simulink model "sim_pos_dist_obs_tie"  (R2020a)
settings: Solver=ode4  StartTime=0.0  StopTime=30.0  FixedStep=0.01  RelTol=1e-3
values from neighbouring files (symbols this model uses):
  alfa_theta = 20    [init_pos_dist_obs_tie.m]
  alfa_theta_obs = 100    [init_pos_dist_obs_tie.m]
  beta1 = 1.2    [init_pos_dist_obs_tie.m]
  beta2 = 0.8    [init_pos_dist_obs_tie.m]
  delta_p_i_0 = zeros(3, NF)    [init_pos_dist_obs_tie.m]
  delta_v_i_0 = zeros(3, NF)    [init_pos_dist_obs_tie.m]
  dp_aa_t = 0.2 * ones(3, 5) + ( 1.0 - 0.2 ) * rand(3, 5)    [init_pos_dist_obs_tie.m]
  dp_ff_t = [ 0.4 * ones(1, 5) + ( 1.0 - 0.4 ) * rand(1, 5);                      0.4 * ones(1, 5) + ( 1.0 - 0.4 ) * rand(1, 5);                      0.2 * ones(1, 5) + ( 0.6 - 0.2 ) * rand(1, 5) ]    [init_pos_dist_obs_tie.m]
  dp_phi_t = ( - pi / 2 ) * ones(3, 5) + ( pi / 2 - ( - pi / 2 ) ) * rand(3, 5)    [init_pos_dist_obs_tie.m]
  ell1v = [2 * (Lv ^ (1/3)); 2 * (Lv ^ (1/3)); 2 * (Lv ^ (1/3))]    [init_pos_dist_obs_tie.m]
  ell2v = [1.5 * (Lv ^ (2/3)); 1.5 * (Lv ^ (2/3)); 1.5 * (Lv ^ (2/3))]    [init_pos_dist_obs_tie.m]
  ell3v = [1.1 * Lv; 1.1 * Lv; 1.1 * Lv]    [init_pos_dist_obs_tie.m]
  etai_0 = zeros(3,5)    [init_pos_dist_obs_tie.m]
  kai1v = [20; 20; 20]    [init_pos_dist_obs_tie.m]
  kai2v = [20; 20; 20]    [init_pos_dist_obs_tie.m]
  kai3v = [20; 20; 20]    [init_pos_dist_obs_tie.m]
  kai_1_t = 0.02    [init_pos_dist_obs_tie.m]
  kai_3_t = 0.1    [init_pos_dist_obs_tie.m]
  kai_chi_1 = diag([6; 6; 6])    [init_pos_dist_obs_tie.m]
  kai_chi_2 = diag([6; 6; 6])    [init_pos_dist_obs_tie.m]
  kai_u_1 = diag([8; 8; 8])    [init_pos_dist_obs_tie.m]
  kai_u_2 = diag([8; 8; 8])    [init_pos_dist_obs_tie.m]
  ksii_0 = zeros(3,5)    [init_pos_dist_obs_tie.m]
  l1v = diag([20; 20; 20])    [init_pos_dist_obs_tie.m]
  l2v = diag([30; 30; 30])    [init_pos_dist_obs_tie.m]
  mass_i = zeros(1,NF)    [init_pos_dist_obs_tie.m]
  Mii = diag([1;0;0;0;1])    [init_pos_dist_obs_tie.m]
  pos0 = zeros(3, 1)    [init_pos_dist_obs_tie.m]
  PZ0 = P0(3)    [init_pos_dist_obs_tie.m]
  PZ1 = 10    [init_pos_dist_obs_tie.m]
  Qci_init = repmat([1;0;0;0],1,NF)    [init_pos_dist_obs_tie.m]
  R0 = 4    [init_pos_dist_obs_tie.m]
  R1 = 8    [init_pos_dist_obs_tie.m]
  Rx2 = 10    [init_pos_dist_obs_tie.m]
  Ry2 = 6    [init_pos_dist_obs_tie.m]
  Rz2 = 4    [init_pos_dist_obs_tie.m]
  T0 = 0    [init_pos_dist_obs_tie.m]
  T1 = tseq1    (= 10)    [init_pos_dist_obs_tie.m]
  T12 = tseq1 + tseq12    (= 20)    [init_pos_dist_obs_tie.m]
  T2 = tseq1 + tseq12 + tseq2    (= 30)    [init_pos_dist_obs_tie.m]
  theta0 = ( 2 / 5 ) * pi    (= 1.25663706144)    [init_pos_dist_obs_tie.m]
  vel0 = zeros(3, 1)    [init_pos_dist_obs_tie.m]
  Wij = [0,0,1,0,0;              0,0,1,1,0;              1,0,0,0,1;              0,1,1,0,0;              0,0,1,0,0]    [init_pos_dist_obs_tie.m]
  X1 = 8    [init_pos_dist_obs_tie.m]
  X2 = 2    [init_pos_dist_obs_tie.m]
  X3 = 3    [init_pos_dist_obs_tie.m]
  Y1 = 10    [init_pos_dist_obs_tie.m]
  Y2 = 2    [init_pos_dist_obs_tie.m]
  Y3 = 4    [init_pos_dist_obs_tie.m]
  Z1 = 4    [init_pos_dist_obs_tie.m]
  Z2 = -6    [init_pos_dist_obs_tie.m]
  Z3 = 2    [init_pos_dist_obs_tie.m]
undefined symbols (not defined in the file or in its folder): cal_frac_squ, p_beta1, p_beta2, p_dbeta1, p_dbeta2, p_gamma1_pos, p_gamma1_vel, p_gamma2_pos, p_gamma2_vel, p_m_1, p_m_2, p_m_3, q_beta1, q_beta2, q_dbeta1, q_dbeta2, q_gamma1_pos, q_gamma1_vel, q_gamma2_pos, q_gamma2_vel, q_m_1, q_m_2, q_m_3
(part 4 of 4)

== matlab function sim_pos_dist_obs_tie/virtual velocity tracking item agent 1 ==
  data: kai_chi_1 input; chi_1 output; kai_chi_2 input; theta_err_ksi_1_vec input; theta_err_ksi_2_vec input
function chi_1 = fcn(kai_chi_1, kai_chi_2, theta_err_ksi_1_vec, theta_err_ksi_2_vec)
%%%% 固定时间虚拟速度控制量chi
iiuav = 1;
chi_1 = -kai_chi_1 * theta_err_ksi_1_vec(:,iiuav) - kai_chi_2 * theta_err_ksi_2_vec(:,iiuav);

== matlab function sim_pos_dist_obs_tie/virtual velocity tracking item agent 2 ==
  data: kai_chi_1 input; chi_2 output; kai_chi_2 input; theta_err_ksi_1_vec input; theta_err_ksi_2_vec input
function chi_2 = fcn(kai_chi_1, kai_chi_2, theta_err_ksi_1_vec, theta_err_ksi_2_vec)
%%%% 固定时间虚拟速度控制量chi
iiuav = 2;
chi_2 = -kai_chi_1 * theta_err_ksi_1_vec(:,iiuav) - kai_chi_2 * theta_err_ksi_2_vec(:,iiuav);

== matlab function sim_pos_dist_obs_tie/virtual velocity tracking item agent 3 ==
  data: kai_chi_1 input; chi_3 output; kai_chi_2 input; theta_err_ksi_1_vec input; theta_err_ksi_2_vec input
function chi_3 = fcn(kai_chi_1, kai_chi_2, theta_err_ksi_1_vec, theta_err_ksi_2_vec)
%%%% 固定时间虚拟速度控制量chi
iiuav = 3;
chi_3 = -kai_chi_1 * theta_err_ksi_1_vec(:,iiuav) - kai_chi_2 * theta_err_ksi_2_vec(:,iiuav);

== matlab function sim_pos_dist_obs_tie/virtual velocity tracking item agent 4 ==
  data: kai_chi_1 input; chi_4 output; kai_chi_2 input; theta_err_ksi_1_vec input; theta_err_ksi_2_vec input
function chi_4 = fcn(kai_chi_1, kai_chi_2, theta_err_ksi_1_vec, theta_err_ksi_2_vec)
%%%% 固定时间虚拟速度控制量chi
iiuav = 4;
chi_4 = -kai_chi_1 * theta_err_ksi_1_vec(:,iiuav) - kai_chi_2 * theta_err_ksi_2_vec(:,iiuav);

== matlab function sim_pos_dist_obs_tie/virtual velocity tracking item agent 5 ==
  data: kai_chi_1 input; chi_5 output; kai_chi_2 input; theta_err_ksi_1_vec input; theta_err_ksi_2_vec input
function chi_5 = fcn(kai_chi_1, kai_chi_2, theta_err_ksi_1_vec, theta_err_ksi_2_vec)
%%%% 固定时间虚拟速度控制量chi
iiuav = 5;
chi_5 = -kai_chi_1 * theta_err_ksi_1_vec(:,iiuav) - kai_chi_2 * theta_err_ksi_2_vec(:,iiuav);

== matlab function sim_pos_dist_obs_tie/combine chi ==
  data: chi_1 input; chi_2 input; chi_3 input; chi_4 input; chi_5 input; chi_vec output
function chi_vec  = fcn(chi_1, chi_2, chi_3, chi_4, chi_5)
%%%% 合并领导者位置观测器输出结果
chi_vec = [chi_1(:), chi_2(:), chi_3(:), chi_4(:), chi_5(:)];

== matlab function sim_pos_dist_obs_tie/generate translational disturbance agent 1 ==
  data: dp_aa_t input; dp_ff_t input; dp_phi_t input; dp_1 output; t input
function dp_1 = fcn(dp_aa_t, dp_ff_t, dp_phi_t, t)
%%%% 平移动力学方程中的扰动项设置
epsil_t = zeros(3, 1);

for kk = 1:5
    epsil_t = epsil_t + dp_aa_t(:, kk) .* sin( 2 * pi * dp_ff_t(:, kk) * t + dp_phi_t(:, kk) );
end

dp_1 = [ epsil_t(1) + 1.6 * sin( 0.4 * t ) + 2.0 * cos( 0.5 * t ) + 1.4 * sin( 0.7 * t ) ...
                + 4 * exp( -0.1 * t ) * sin( 0.8 * t ) + 3 / ( 1 + exp( -0.2 * ( t - 15 ) ) ); ...
                epsil_t(2) + 1.2 * sin( 0.2 * t ) + 3 * cos( 0.4 * t ) + 0.8 * sin( 0.6 * t ) ...
                + 2 * exp( -0.15 * t ) * cos( 1.2 * t ) + 3 / ( 1 + exp( -0.3 * ( t - 25 ) ) ); ...
                epsil_t(3) + 1.8 * sin( 0.2 * t ) + 1.6 * sin( 0.3 * t ) + 1.6 * cos( 0.4 * t ) ...
                + 4 * exp( -0.05 * t ) * sin( 0.5 * t + pi / 4 ) + 3 / ( 1 + exp( -0.5 * ( t - 20 ) ) ) ];

== matlab function sim_pos_dist_obs_tie/cal virtual velocity control error phi ==
  data: err_eta_vec input; chi_vec input; phi_vec output
function phi_vec  = fcn(err_eta_vec, chi_vec)
%%%% 合并领导者位置观测器输出结果
phi_vec = zeros(3,5);
for iiuav = 1:5
    phi_vec(:,iiuav) = err_eta_vec(:,iiuav) - chi_vec(:,iiuav);
end

== matlab function sim_pos_dist_obs_tie/cal abs 11 ==
  data: x input; y output
function y = fcn(x)
y = abs(x(:));

== matlab function sim_pos_dist_obs_tie/cal abs 12 ==
  data: x input; y output
function y = fcn(x)
y = abs(x(:));

== matlab function sim_pos_dist_obs_tie/choose ksi_est_err 11 ==
  data: x input; y output
function y = fcn(x)
iiuav = 1;
y = x(:,iiuav);

== matlab function sim_pos_dist_obs_tie/choose ksi_est_err 12 ==
  data: x input; y output
function y = fcn(x)
iiuav = 1;
y = x(:,iiuav);

== matlab function sim_pos_dist_obs_tie/trans to column10 ==
  data: x input; y output
function y = fcn(x)
y = x(:);

== matlab function sim_pos_dist_obs_tie/trans to column11 ==
  data: x input; y output
function y = fcn(x)
y = x(:);

== matlab function sim_pos_dist_obs_tie/cal d_theta_err_ksi agent 1 ==
  data: alfa_theta input; beta1 input; d_theta_err_ksi_1_1 output; beta2 input; d_err_ksi_squ_1_node_1 input; d_err_ksi_squ_2_node_1 input; err_ksi_squ_1_node_1 input; err_ksi_squ_2_node_1 input; err_ksi_vec input; d_theta_err_ksi_2_1 output; err_eta_vec input
function [d_theta_err_ksi_1_1, d_theta_err_ksi_2_1] = fcn(alfa_theta, beta1, beta2, d_err_ksi_squ_1_node_1, d_err_ksi_squ_2_node_1, ...
                                                                                                        err_ksi_squ_1_node_1, err_ksi_squ_2_node_1, err_ksi_vec, err_eta_vec)
%%%% 计算平滑递增函数的导数
iiuav = 1;
kk_alfa = alfa_theta;
d_theta_err_ksi_1_1 = ( beta1 .* d_err_ksi_squ_1_node_1(:) .* sign(err_ksi_vec(:,iiuav)) .* ( -1 + 2 ./ ( 1 + exp( -kk_alfa .* err_ksi_vec(:,iiuav) ) ) ) + ...
                                            err_ksi_squ_1_node_1(:) .* ( 2 .* kk_alfa .* exp( -kk_alfa .* err_ksi_vec(:,iiuav) ) ./ ( ( 1 + exp( -kk_alfa .* err_ksi_vec(:,iiuav) ) ) .^ 2) ) ) ...
                                            .* err_eta_vec(:,iiuav);
d_theta_err_ksi_2_1 = ( beta2 .* d_err_ksi_squ_2_node_1(:) .* sign(err_ksi_vec(:,iiuav)) .* ( -1 + 2 ./ ( 1 + exp( -kk_alfa .* err_ksi_vec(:,iiuav) ) ) ) + ...
                                            err_ksi_squ_2_node_1(:) .* ( 2 .* kk_alfa .* exp( -kk_alfa .* err_ksi_vec(:,iiuav) ) ./ ( ( 1 + exp( -kk_alfa .* err_ksi_vec(:,iiuav) ) ) .^ 2) ) ) ...
                                            .* err_eta_vec(:,iiuav);

== matlab function sim_pos_dist_obs_tie/cal abs 13 ==
  data: x input; y output
function y = fcn(x)
y = abs(x(:));

== matlab function sim_pos_dist_obs_tie/cal abs 14 ==
  data: x input; y output
function y = fcn(x)
y = abs(x(:));

== matlab function sim_pos_dist_obs_tie/cal d_theta_err_ksi agent 2 ==
  data: alfa_theta input; beta1 input; d_theta_err_ksi_1_2 output; beta2 input; d_err_ksi_squ_1_node_2 input; d_err_ksi_squ_2_node_2 input; err_ksi_squ_1_node_2 input; err_ksi_squ_2_node_2 input; err_ksi_vec input; d_theta_err_ksi_2_2 output; err_eta_vec input
function [d_theta_err_ksi_1_2, d_theta_err_ksi_2_2] = fcn(alfa_theta, beta1, beta2, d_err_ksi_squ_1_node_2, d_err_ksi_squ_2_node_2, ...
                                                                                                        err_ksi_squ_1_node_2, err_ksi_squ_2_node_2, err_ksi_vec, err_eta_vec)
%%%% 计算平滑递增函数的导数
iiuav = 2;
kk_alfa = alfa_theta;
d_theta_err_ksi_1_2 = ( beta1 .* d_err_ksi_squ_1_node_2(:) .* sign(err_ksi_vec(:,iiuav)) .* ( -1 + 2 ./ ( 1 + exp( -kk_alfa .* err_ksi_vec(:,iiuav) ) ) ) + ...
                                            err_ksi_squ_1_node_2(:) .* ( 2 .* kk_alfa .* exp( -kk_alfa .* err_ksi_vec(:,iiuav) ) ./ ( ( 1 + exp( -kk_alfa .* err_ksi_vec(:,iiuav) ) ) .^ 2) ) ) ...
                                            .* err_eta_vec(:,iiuav);
d_theta_err_ksi_2_2 = ( beta2 .* d_err_ksi_squ_2_node_2(:) .* sign(err_ksi_vec(:,iiuav)) .* ( -1 + 2 ./ ( 1 + exp( -kk_alfa .* err_ksi_vec(:,iiuav) ) ) ) + ...
                                            err_ksi_squ_2_node_2(:) .* ( 2 .* kk_alfa .* exp( -kk_alfa .* err_ksi_vec(:,iiuav) ) ./ ( ( 1 + exp( -kk_alfa .* err_ksi_vec(:,iiuav) ) ) .^ 2) ) ) ...
                                            .* err_eta_vec(:,iiuav);

== matlab function sim_pos_dist_obs_tie/generate translational disturbance agent 2 ==
  data: dp_aa_t input; dp_ff_t input; dp_phi_t input; dp_2 output; t input
function dp_2 = fcn(dp_aa_t, dp_ff_t, dp_phi_t, t)
%%%% 平移动力学方程中的扰动项设置
epsil_t = zeros(3, 1);

for kk = 1:5
    epsil_t = epsil_t + dp_aa_t(:, kk) .* sin( 2 * pi * dp_ff_t(:, kk) * t + dp_phi_t(:, kk) );
end

dp_2 = [ epsil_t(1) + 1.6 * sin( 0.2 * t ) + 2.0 * cos( 0.3 * t ) + 1.4 * sin( 0.5 * t ) ...
                + 4 * exp( -0.1 * t ) * sin( 0.5 * t ) + 3 / ( 1 + exp( -0.2 * ( t - 15 ) ) ); ...
                epsil_t(2) + 1.2 * sin( 0.1 * t ) + 3 * cos( 0.2 * t ) + 0.8 * sin( 0.4 * t ) ...
                + 2 * exp( -0.15 * t ) * cos( 0.6 * t ) + 3 / ( 1 + exp( -0.3 * ( t - 25 ) ) ); ...
                epsil_t(3) + 1.8 * sin( 0.1 * t ) + 1.6 * sin( 0.2 * t ) + 1.6 * cos( 0.3 * t ) ...
                + 4 * exp( -0.05 * t ) * sin( 0.4 * t + pi / 4 ) + 3 / ( 1 + exp( -0.5 * ( t - 20 ) ) ) ];

== matlab function sim_pos_dist_obs_tie/choose ksi_est_err 13 ==
  data: x input; y output
function y = fcn(x)
iiuav = 2;
y = x(:,iiuav);

== matlab function sim_pos_dist_obs_tie/choose ksi_est_err 14 ==
  data: x input; y output
function y = fcn(x)
iiuav = 2;
y = x(:,iiuav);

== matlab function sim_pos_dist_obs_tie/trans to column12 ==
  data: x input; y output
function y = fcn(x)
y = x(:);

== matlab function sim_pos_dist_obs_tie/trans to column13 ==
  data: x input; y output
function y = fcn(x)
y = x(:);

== matlab function sim_pos_dist_obs_tie/cal abs 15 ==
  data: x input; y output
function y = fcn(x)
y = abs(x(:));

== matlab function sim_pos_dist_obs_tie/cal abs 16 ==
  data: x input; y output
function y = fcn(x)
y = abs(x(:));

== matlab function sim_pos_dist_obs_tie/cal d_theta_err_ksi agent 3 ==
  data: alfa_theta input; beta1 input; d_theta_err_ksi_1_3 output; beta2 input; d_err_ksi_squ_1_node_3 input; d_err_ksi_squ_2_node_3 input; err_ksi_squ_1_node_3 input; err_ksi_squ_2_node_3 input; err_ksi_vec input; d_theta_err_ksi_2_3 output; err_eta_vec input
function [d_theta_err_ksi_1_3, d_theta_err_ksi_2_3] = fcn(alfa_theta, beta1, beta2, d_err_ksi_squ_1_node_3, d_err_ksi_squ_2_node_3, ...
                                                                                                        err_ksi_squ_1_node_3, err_ksi_squ_2_node_3, err_ksi_vec, err_eta_vec)
%%%% 计算平滑递增函数的导数
iiuav = 3;
kk_alfa = alfa_theta;
d_theta_err_ksi_1_3 = ( beta1 .* d_err_ksi_squ_1_node_3(:) .* sign(err_ksi_vec(:,iiuav)) .* ( -1 + 2 ./ ( 1 + exp( -kk_alfa .* err_ksi_vec(:,iiuav) ) ) ) + ...
                                            err_ksi_squ_1_node_3(:) .* ( 2 .* kk_alfa .* exp( -kk_alfa .* err_ksi_vec(:,iiuav) ) ./ ( ( 1 + exp( -kk_alfa .* err_ksi_vec(:,iiuav) ) ) .^ 2) ) ) ...
                                            .* err_eta_vec(:,iiuav);
d_theta_err_ksi_2_3 = ( beta2 .* d_err_ksi_squ_2_node_3(:) .* sign(err_ksi_vec(:,iiuav)) .* ( -1 + 2 ./ ( 1 + exp( -kk_alfa .* err_ksi_vec(:,iiuav) ) ) ) + ...
                                            err_ksi_squ_2_node_3(:) .* ( 2 .* kk_alfa .* exp( -kk_alfa .* err_ksi_vec(:,iiuav) ) ./ ( ( 1 + exp( -kk_alfa .* err_ksi_vec(:,iiuav) ) ) .^ 2) ) ) ...
                                            .* err_eta_vec(:,iiuav);

== matlab function sim_pos_dist_obs_tie/choose ksi_est_err 15 ==
  data: x input; y output
function y = fcn(x)
iiuav = 3;
y = x(:,iiuav);

== matlab function sim_pos_dist_obs_tie/choose ksi_est_err 16 ==
  data: x input; y output
function y = fcn(x)
iiuav = 3;
y = x(:,iiuav);

== matlab function sim_pos_dist_obs_tie/trans to column14 ==
  data: x input; y output
function y = fcn(x)
y = x(:);

== matlab function sim_pos_dist_obs_tie/trans to column15 ==
  data: x input; y output
function y = fcn(x)
y = x(:);

== matlab function sim_pos_dist_obs_tie/cal abs 17 ==
  data: x input; y output
function y = fcn(x)
y = abs(x(:));

== matlab function sim_pos_dist_obs_tie/cal abs 18 ==
  data: x input; y output
function y = fcn(x)
y = abs(x(:));

== matlab function sim_pos_dist_obs_tie/generate translational disturbance agent 3 ==
  data: dp_aa_t input; dp_ff_t input; dp_phi_t input; dp_3 output; t input
function dp_3 = fcn(dp_aa_t, dp_ff_t, dp_phi_t, t)
%%%% 平移动力学方程中的扰动项设置
epsil_t = zeros(3, 1);

for kk = 1:5
    epsil_t = epsil_t + dp_aa_t(:, kk) .* sin( 2 * pi * dp_ff_t(:, kk) * t + dp_phi_t(:, kk) );
end

dp_3 = [ epsil_t(1) + 1.6 * sin( 0.2 * t ) + 2.0 * cos( 0.3 * t ) + 1.4 * sin( 0.5 * t ) ...
                + 4 * exp( -0.1 * t ) * sin( 0.5 * t ) + 3 / ( 1 + exp( -0.2 * ( t - 15 ) ) ); ...
                epsil_t(2) + 1.2 * sin( 0.1 * t ) + 3 * cos( 0.2 * t ) + 0.8 * sin( 0.4 * t ) ...
                + 2 * exp( -0.15 * t ) * cos( 0.6 * t ) + 3 / ( 1 + exp( -0.3 * ( t - 25 ) ) ); ...
                epsil_t(3) + 1.8 * sin( 0.1 * t ) + 1.6 * sin( 0.2 * t ) + 1.6 * cos( 0.3 * t ) ...
                + 4 * exp( -0.05 * t ) * sin( 0.4 * t + pi / 4 ) + 3 / ( 1 + exp( -0.5 * ( t - 20 ) ) ) ];

== matlab function sim_pos_dist_obs_tie/cal d_theta_err_ksi agent 4 ==
  data: alfa_theta input; beta1 input; d_theta_err_ksi_1_4 output; beta2 input; d_err_ksi_squ_1_node_4 input; d_err_ksi_squ_2_node_4 input; err_ksi_squ_1_node_4 input; err_ksi_squ_2_node_4 input; err_ksi_vec input; d_theta_err_ksi_2_4 output; err_eta_vec input
function [d_theta_err_ksi_1_4, d_theta_err_ksi_2_4] = fcn(alfa_theta, beta1, beta2, d_err_ksi_squ_1_node_4, d_err_ksi_squ_2_node_4, ...
                                                                                                        err_ksi_squ_1_node_4, err_ksi_squ_2_node_4, err_ksi_vec, err_eta_vec)
%%%% 计算平滑递增函数的导数
iiuav = 4;
kk_alfa = alfa_theta;
d_theta_err_ksi_1_4 = ( beta1 .* d_err_ksi_squ_1_node_4(:) .* sign(err_ksi_vec(:,iiuav)) .* ( -1 + 2 ./ ( 1 + exp( -kk_alfa .* err_ksi_vec(:,iiuav) ) ) ) + ...
                                            err_ksi_squ_1_node_4(:) .* ( 2 .* kk_alfa .* exp( -kk_alfa .* err_ksi_vec(:,iiuav) ) ./ ( ( 1 + exp( -kk_alfa .* err_ksi_vec(:,iiuav) ) ) .^ 2) ) ) ...
                                            .* err_eta_vec(:,iiuav);
d_theta_err_ksi_2_4 = ( beta2 .* d_err_ksi_squ_2_node_4(:) .* sign(err_ksi_vec(:,iiuav)) .* ( -1 + 2 ./ ( 1 + exp( -kk_alfa .* err_ksi_vec(:,iiuav) ) ) ) + ...
                                            err_ksi_squ_2_node_4(:) .* ( 2 .* kk_alfa .* exp( -kk_alfa .* err_ksi_vec(:,iiuav) ) ./ ( ( 1 + exp( -kk_alfa .* err_ksi_vec(:,iiuav) ) ) .^ 2) ) ) ...
                                            .* err_eta_vec(:,iiuav);

== matlab function sim_pos_dist_obs_tie/choose ksi_est_err 17 ==
  data: x input; y output
function y = fcn(x)
iiuav = 4;
y = x(:,iiuav);

== matlab function sim_pos_dist_obs_tie/choose ksi_est_err 18 ==
  data: x input; y output
function y = fcn(x)
iiuav = 4;
y = x(:,iiuav);

== matlab function sim_pos_dist_obs_tie/trans to column16 ==
  data: x input; y output
function y = fcn(x)
y = x(:);

== matlab function sim_pos_dist_obs_tie/trans to column17 ==
  data: x input; y output
function y = fcn(x)
y = x(:);

== matlab function sim_pos_dist_obs_tie/cal abs 19 ==
  data: x input; y output
function y = fcn(x)
y = abs(x(:));

== matlab function sim_pos_dist_obs_tie/cal abs 20 ==
  data: x input; y output
function y = fcn(x)
y = abs(x(:));

== matlab function sim_pos_dist_obs_tie/cal d_theta_err_ksi agent 5 ==
  data: alfa_theta input; beta1 input; d_theta_err_ksi_1_5 output; beta2 input; d_err_ksi_squ_1_node_5 input; d_err_ksi_squ_2_node_5 input; err_ksi_squ_1_node_5 input; err_ksi_squ_2_node_5 input; err_ksi_vec input; d_theta_err_ksi_2_5 output; err_eta_vec input
function [d_theta_err_ksi_1_5, d_theta_err_ksi_2_5] = fcn(alfa_theta, beta1, beta2, d_err_ksi_squ_1_node_5, d_err_ksi_squ_2_node_5, ...
                                                                                                        err_ksi_squ_1_node_5, err_ksi_squ_2_node_5, err_ksi_vec, err_eta_vec)
%%%% 计算平滑递增函数的导数
iiuav = 5;
kk_alfa = alfa_theta;
d_theta_err_ksi_1_5 = ( beta1 .* d_err_ksi_squ_1_node_5(:) .* sign(err_ksi_vec(:,iiuav)) .* ( -1 + 2 ./ ( 1 + exp( -kk_alfa .* err_ksi_vec(:,iiuav) ) ) ) + ...
                                            err_ksi_squ_1_node_5(:) .* ( 2 .* kk_alfa .* exp( -kk_alfa .* err_ksi_vec(:,iiuav) ) ./ ( ( 1 + exp( -kk_alfa .* err_ksi_vec(:,iiuav) ) ) .^ 2) ) ) ...
                                            .* err_eta_vec(:,iiuav);
d_theta_err_ksi_2_5 = ( beta2 .* d_err_ksi_squ_2_node_5(:) .* sign(err_ksi_vec(:,iiuav)) .* ( -1 + 2 ./ ( 1 + exp( -kk_alfa .* err_ksi_vec(:,iiuav) ) ) ) + ...
                                            err_ksi_squ_2_node_5(:) .* ( 2 .* kk_alfa .* exp( -kk_alfa .* err_ksi_vec(:,iiuav) ) ./ ( ( 1 + exp( -kk_alfa .* err_ksi_vec(:,iiuav) ) ) .^ 2) ) ) ...
                                            .* err_eta_vec(:,iiuav);
